simulink model "untitled"  (R2022b)
settings: Solver=FixedStepAuto  StartTime=0.0  StopTime=2  FixedStep=0.01  RelTol=1e-3
undefined symbols (not defined in the file): DiscIntNeverNeededParam
settings Model: Creator=Robert  LastModifiedBy=Robert

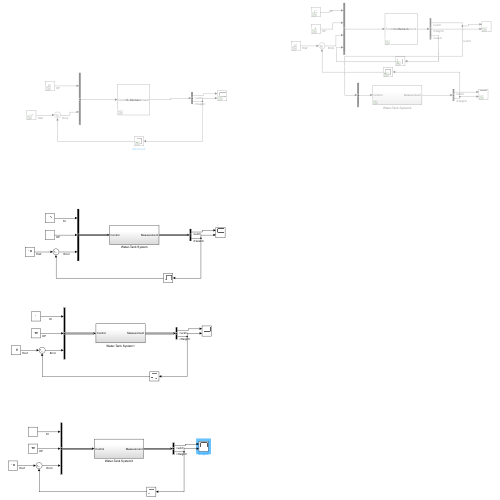
[thumbnail: Simulink's stored preview of the top-level diagram]
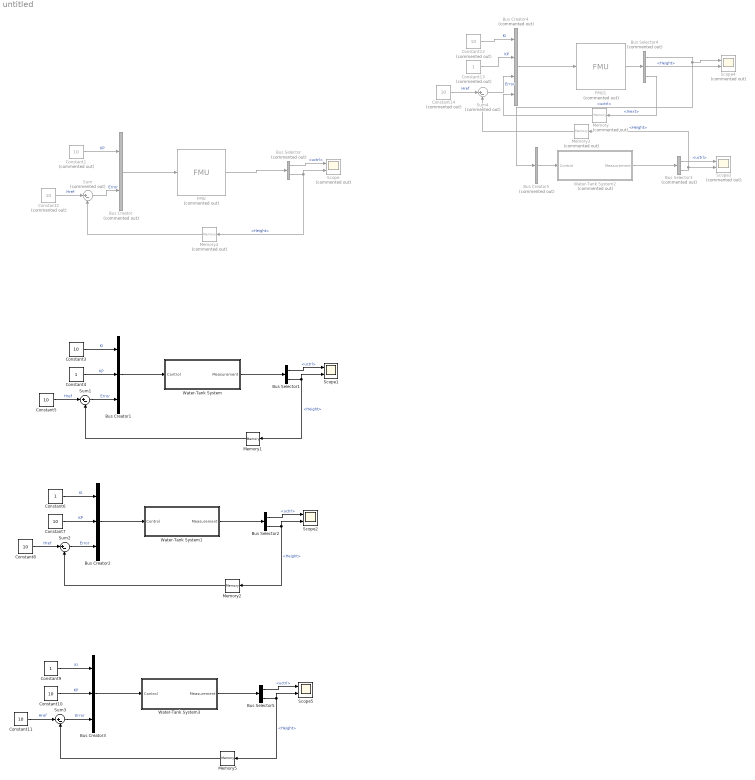
== system untitled ==
  Bus Creator : BusCreator  Commented=on  Inputs=2  OutDataTypeStr=Bus: Control  NonVirtualBus=on
  Bus Creator1 : BusCreator  Inputs=3
  Bus Creator2 : BusCreator  Inputs=3
  Bus Creator3 : BusCreator  Inputs=3
  Bus Creator4 : BusCreator  Commented=on  Inputs=4  OutDataTypeStr=Bus: Control  NonVirtualBus=on
  Bus Creator5 : BusCreator  Commented=on  Inputs=1
  Bus Selector : BusSelector  Commented=on  OutputSignals=uctrl,Height
  Bus Selector1 : BusSelector  OutputSignals=uctrl,Height
  Bus Selector2 : BusSelector  OutputSignals=uctrl,Height
  Bus Selector3 : BusSelector  Commented=on  OutputSignals=uctrl,Height
  Bus Selector4 : BusSelector  Commented=on  OutputSignals=uctrl,Height,Inext
  Bus Selector5 : BusSelector  OutputSignals=uctrl,Height
  Constant{1..2,12,14} (4 alike) : Constant  Commented=on  Value=10
  Constant{3,5,7..8,10..11} (6 alike) : Constant  Value=10
  Constant13 : Constant  Commented=on
  Constant4 : Constant
  Constant6 : Constant
  Constant9 : Constant
  FMU : FMU  Commented=on  FMUName=rlwatertank.fmu  FMUMode=CoSimulation  FMUCreateBusObject=off
      mask Type: rlwatertank [Co-Simulation, v2.0]
      mask Display:
      | disp('rlwatertank');
      | port_label('output',1,'Measurement');
      | port_label('input',1,'Control');
  FMU1 : FMU  Commented=on  FMUName=rlwatertank.fmu  FMUMode=CoSimulation  FMUIsToleranceUsed=on  FMUToleranceValue=1E-06  FMUSampleTime=0.01  FMUCreateBusObject=off
      mask Type: rlwatertank [Co-Simulation, v2.0]
      mask Display:
      | disp('rlwatertank');
      | port_label('output',1,'Measurement');
      | port_label('input',1,'Control');
  Memory : Memory  Commented=on
  Memory1 : Memory
  Memory2 : Memory
  Memory3 : Memory  Commented=on
  Memory4 : Memory  Commented=on
  Memory5 : Memory
  Scope : Scope  Commented=on  NumInputPorts=2
  Scope1 : Scope  NumInputPorts=2
  Scope2 : Scope  NumInputPorts=2
  Scope3 : Scope  Commented=on  NumInputPorts=2
  Scope4 : Scope  Commented=on  NumInputPorts=2
  Scope5 : Scope  NumInputPorts=2
  Sum : Sum  Commented=on  Inputs=|+-
  Sum1 : Sum  Inputs=|+-
  Sum2 : Sum  Inputs=|+-
  Sum3 : Sum  Inputs=|+-
  Sum4 : Sum  Commented=on  Inputs=|+-
  Water-Tank System : Subsystem
  Water-Tank System1 : Subsystem
  Water-Tank System2 : Subsystem  Commented=on
  Water-Tank System3 : Subsystem
  wires:
  Bus Creator/1 -> FMU/1
  Constant2/1 -> Sum/1  "Href"
  Bus Selector/2 -> Memory4/1, Scope/2  "<Height>"
  Bus Selector/1 -> Scope/1  "<uctrl>"
  Memory1/1 -> Sum1/2
  Bus Selector1/1 -> Scope1/1  "<uctrl>"
  Bus Selector1/2 -> Memory1/1, Scope1/2  "<Height>"
  Water-Tank System/1(Measurement) -> Bus Selector1/1
  Bus Creator1/1 -> Water-Tank System/1(Control)
  Sum1/1 -> Bus Creator1/3  "Error"
  Constant4/1 -> Bus Creator1/2  "KP"
  Constant5/1 -> Sum1/1  "Href"
  Constant3/1 -> Bus Creator1/1  "KI"
  FMU/1 -> Bus Selector/1
  Constant6/1 -> Bus Creator2/1  "KI"
  Constant8/1 -> Sum2/1  "Href"
  Constant7/1 -> Bus Creator2/2  "KP"
  Sum2/1 -> Bus Creator2/3  "Error"
  Bus Creator2/1 -> Water-Tank System1/1(Control)
  Water-Tank System1/1(Measurement) -> Bus Selector2/1
  Bus Selector2/2 -> Scope2/2, Memory2/1  "<Height>"
  Bus Selector2/1 -> Scope2/1  "<uctrl>"
  Memory2/1 -> Sum2/2
  Water-Tank System2/1(Measurement) -> Bus Selector3/1
  Bus Selector3/2 -> Scope3/2, Memory3/1  "<Height>"
  Bus Selector3/1 -> Scope3/1  "<uctrl>"
  FMU1/1 -> Bus Selector4/1
  Bus Selector4/1 -> Bus Creator5/1, Scope4/1  "<uctrl>"
  Bus Selector4/2 -> Scope4/2  "<Height>"
  Constant14/1 -> Sum4/1  "Href"
  Sum4/1 -> Bus Creator4/3  "Error"
  Constant13/1 -> Bus Creator4/2  "KP"
  Constant12/1 -> Bus Creator4/1  "KI"
  Bus Creator4/1 -> FMU1/1
  Bus Creator5/1 -> Water-Tank System2/1(Control)
  Memory4/1 -> Sum/2
  Memory3/1 -> Sum4/2
  Bus Selector4/3 -> Memory/1  "<Inext>"
  Memory/1 -> Bus Creator4/4
  Constant1/1 -> Bus Creator/1  "KP"
  Sum/1 -> Bus Creator/2  "Error"
  Constant10/1 -> Bus Creator3/2  "KP"
  Memory5/1 -> Sum3/2
  Constant11/1 -> Sum3/1  "Href"
  Bus Creator3/1 -> Water-Tank System3/1(Control)
  Bus Selector5/1 -> Scope5/1  "<uctrl>"
  Water-Tank System3/1(Measurement) -> Bus Selector5/1
  Sum3/1 -> Bus Creator3/3  "Error"
  Bus Selector5/2 -> Scope5/2, Memory5/1  "<Height>"
  Constant9/1 -> Bus Creator3/1  "KI"

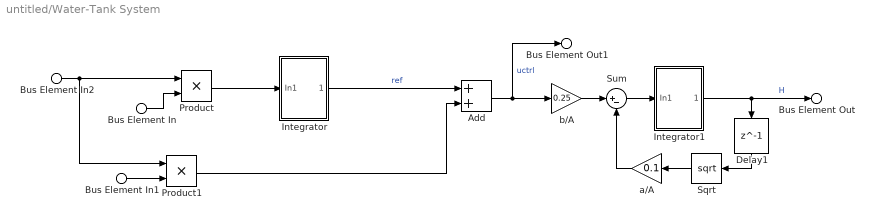
== system untitled/Water-Tank System ==
  Bus Element In2 : Inport  PortName=Control  Element=Error
  Bus Element In : Inport  PortName=Control  Element=KI
  Bus Element In1 : Inport  PortName=Control  Element=KP
  Add : Sum
  Delay1 : Delay  DelayLength=1
  Integrator : Subsystem
  Integrator1 : Subsystem
  Product : Product
  Product1 : Product
  Sqrt : Sqrt  OutputSignalType=real
  Sum : Sum  Inputs=|+-  SaturateOnIntegerOverflow=on
  a/A : Gain  Gain=0.1  SaturateOnIntegerOverflow=on  OutDataTypeStr=Inherit: Same as input  ParamDataTypeStr=Inherit: Same as input
  b/A : Gain  Gain=0.25  SaturateOnIntegerOverflow=on  OutDataTypeStr=Inherit: Same as input  ParamDataTypeStr=Inherit: Same as input
  Bus Element Out : Outport  PortName=Measurement  Element=Height
  Bus Element Out1 : Outport  PortName=Measurement  Element=uctrl
  wires:
  Bus Element In2/1 -> Product1/1, Product/1
  Bus Element In/1 -> Product/2
  Product1/1 -> Add/2
  Bus Element In1/1 -> Product1/2
  Sum/1 -> Integrator1/1(In1)
  Integrator/1(Out1) -> Add/1  "ref"
  a/A/1 -> Sum/2
  b/A/1 -> Sum/1
  Add/1 -> Bus Element Out1/1, b/A/1  "uctrl"
  Integrator1/1(Out1) -> Bus Element Out/1, Delay1/1  "H"
  Sqrt/1 -> a/A/1
  Product/1 -> Integrator/1(In1)
  Delay1/1 -> Sqrt/1

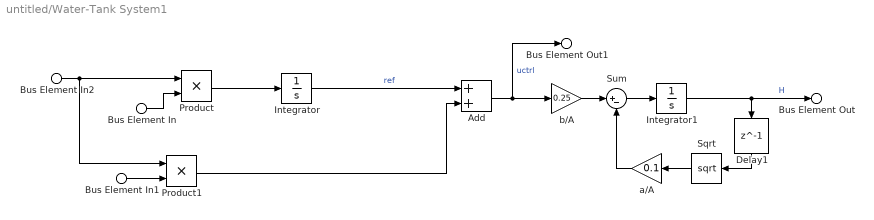
== system untitled/Water-Tank System1 ==
  Bus Element In2 : Inport  PortName=Control  Element=Error
  Bus Element In : Inport  PortName=Control  Element=KI
  Bus Element In1 : Inport  PortName=Control  Element=KP
  Add : Sum
  Delay1 : Delay  DelayLength=1
  Integrator : Integrator
  Integrator1 : Integrator  LimitOutput=on  LowerSaturationLimit=0
  Product : Product
  Product1 : Product
  Sqrt : Sqrt  OutputSignalType=real
  Sum : Sum  Inputs=|+-  SaturateOnIntegerOverflow=on
  a/A : Gain  Gain=0.1  SaturateOnIntegerOverflow=on  OutDataTypeStr=Inherit: Same as input  ParamDataTypeStr=Inherit: Same as input
  b/A : Gain  Gain=0.25  SaturateOnIntegerOverflow=on  OutDataTypeStr=Inherit: Same as input  ParamDataTypeStr=Inherit: Same as input
  Bus Element Out : Outport  PortName=Measurement  Element=Height
  Bus Element Out1 : Outport  PortName=Measurement  Element=uctrl
  wires:
  Delay1/1 -> Sqrt/1
  Product/1 -> Integrator/1
  Sqrt/1 -> a/A/1
  Integrator1/1 -> Delay1/1, Bus Element Out/1  "H"
  Add/1 -> b/A/1, Bus Element Out1/1  "uctrl"
  b/A/1 -> Sum/1
  a/A/1 -> Sum/2
  Integrator/1 -> Add/1  "ref"
  Sum/1 -> Integrator1/1
  Bus Element In1/1 -> Product1/2
  Product1/1 -> Add/2
  Bus Element In/1 -> Product/2
  Bus Element In2/1 -> Product/1, Product1/1

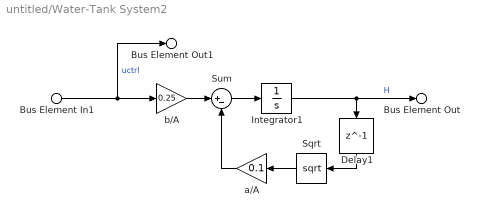
== system untitled/Water-Tank System2 ==
  Bus Element In1 : Inport  PortName=Control  Element=uctrl
  Delay1 : Delay  DelayLength=1
  Integrator1 : Integrator  LimitOutput=on  LowerSaturationLimit=0
  Sqrt : Sqrt  OutputSignalType=real
  Sum : Sum  Inputs=|+-  SaturateOnIntegerOverflow=on
  a/A : Gain  Gain=0.1  SaturateOnIntegerOverflow=on  OutDataTypeStr=Inherit: Same as input  ParamDataTypeStr=Inherit: Same as input
  b/A : Gain  Gain=0.25  SaturateOnIntegerOverflow=on  OutDataTypeStr=Inherit: Same as input  ParamDataTypeStr=Inherit: Same as input
  Bus Element Out : Outport  PortName=Measurement  Element=Height
  Bus Element Out1 : Outport  PortName=Measurement  Element=uctrl
  wires:
  Delay1/1 -> Sqrt/1
  Sqrt/1 -> a/A/1
  Integrator1/1 -> Delay1/1, Bus Element Out/1  "H"
  Bus Element In1/1 -> b/A/1, Bus Element Out1/1  "uctrl"
  b/A/1 -> Sum/1
  a/A/1 -> Sum/2
  Sum/1 -> Integrator1/1

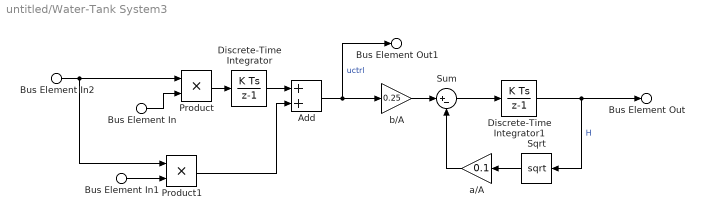
== system untitled/Water-Tank System3 ==
  Bus Element In2 : Inport  PortName=Control  Element=Error
  Bus Element In : Inport  PortName=Control  Element=KI
  Bus Element In1 : Inport  PortName=Control  Element=KP
  Add : Sum
  Discrete-Time Integrator : DiscreteIntegrator  SampleTime=-1  ICPrevOutput=DiscIntNeverNeededParam  ICPrevScaledInput=DiscIntNeverNeededParam
  Discrete-Time Integrator1 : DiscreteIntegrator  InitialCondition=3  SampleTime=-1  ICPrevOutput=DiscIntNeverNeededParam  ICPrevScaledInput=DiscIntNeverNeededParam
  Product : Product
  Product1 : Product
  Sqrt : Sqrt  OutputSignalType=real
  Sum : Sum  Inputs=|+-  SaturateOnIntegerOverflow=on
  a/A : Gain  Gain=0.1  SaturateOnIntegerOverflow=on  OutDataTypeStr=Inherit: Same as input  ParamDataTypeStr=Inherit: Same as input
  b/A : Gain  Gain=0.25  SaturateOnIntegerOverflow=on  OutDataTypeStr=Inherit: Same as input  ParamDataTypeStr=Inherit: Same as input
  Bus Element Out : Outport  PortName=Measurement  Element=Height
  Bus Element Out1 : Outport  PortName=Measurement  Element=uctrl
  wires:
  Discrete-Time Integrator/1 -> Add/1
  Discrete-Time Integrator1/1 -> Bus Element Out/1, Sqrt/1  "H"
  a/A/1 -> Sum/2
  Sum/1 -> Discrete-Time Integrator1/1
  Sqrt/1 -> a/A/1
  Product/1 -> Discrete-Time Integrator/1
  Add/1 -> Bus Element Out1/1, b/A/1  "uctrl"
  Bus Element In1/1 -> Product1/2
  Bus Element In/1 -> Product/2
  Bus Element In2/1 -> Product1/1, Product/1
  Product1/1 -> Add/2
  b/A/1 -> Sum/1

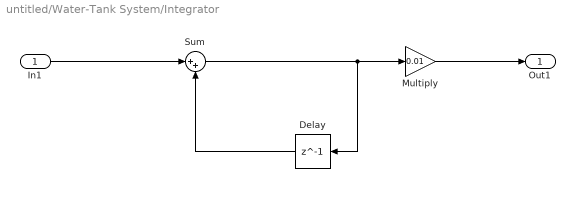
== system untitled/Water-Tank System/Integrator ==
  In1 : Inport
  Delay : Delay  DelayLength=1
  Multiply : Gain  Gain=0.01
  Sum : Sum  Inputs=|++
  Out1 : Outport
  wires:
  In1/1 -> Sum/1
  Delay/1 -> Sum/2
  Sum/1 -> Delay/1, Multiply/1
  Multiply/1 -> Out1/1

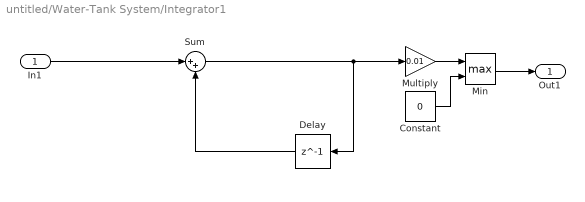
== system untitled/Water-Tank System/Integrator1 ==
  In1 : Inport
  Constant : Constant  Value=0
  Delay : Delay  DelayLength=1
  Min : MinMax  Function=max  Inputs=2
  Multiply : Gain  Gain=0.01
  Sum : Sum  Inputs=|++
  Out1 : Outport
  wires:
  In1/1 -> Sum/1
  Delay/1 -> Sum/2
  Sum/1 -> Delay/1, Multiply/1
  Multiply/1 -> Min/1
  Min/1 -> Out1/1
  Constant/1 -> Min/2
